simulink model "Modes_Serial"  (R2022b)
settings: Solver=FixedStepAuto  StartTime=0.0  StopTime=10.0  FixedStep=1e-3  RelTol=1e-3  EnableMultiTasking=on
undefined symbols (not defined in the file): A0, A1, D0, D1, D10, D11, D12, D13, D2, D3, D4, D5, D6, D7, D8, D9, PTA0, PTA1, PTA2, PTB2, PTB23, PTB3, PTB9, PTC16, PTC17, PTC2, PTC3, PTC4, PTD0, PTD1, PTD2, PTD3
libraries: etargetslib x22, frdmk64flib x21
settings Model: ExtModeTrigDuration=5  Creator=haotianxue  LastModifiedBy=kavem
settings OptimizationCC: EnhancedBackFolding=on  PassReuseOutputArgsAs=Individual arguments  ZeroExternalMemoryAtStartup=off  ZeroInternalMemoryAtStartup=off  MaxStackSize=64  OptimizeBlockOrder=speed  DifferentSizesBufferReuse=on  OptimizationCustomize=off  EfficientTunableParamExpr=on
settings DebuggingCC: ParameterTunabilityLossMsg=error  UnconnectedInputMsg=warning  UnconnectedOutputMsg=warning  UnconnectedLineMsg=warning
settings HardwareCC: ProdBitPerPointer=32  ProdBitPerSizeT=32  ProdBitPerPtrDiffT=32  ProdLargestAtomicInteger=Long  ProdLargestAtomicFloat=Double  ProdWordSize=32  ProdHWDeviceType=ARM Compatible->ARM Cortex
settings ModelReferenceCC: EnableRefExpFcnMdlSchedulingChecks=on
settings SFSimCC: MATLABDynamicMemAlloc=off
settings RTWCC: Description=Embedded Coder  SystemTargetFile=ert.tlc  HardwareBoard=NXP FRDM-K64F  TLCOptions="-aInlineSetEventsForThisBaseRateFcn=TLC_FALSE -aSuppressMultiTaskScheduler=TLC_FALSE  -aRateBasedStepFcn=0"  TemplateMakefile=ert_default_tmf  Toolchain=GNU Tools for ARM Embedded Processors  DLArmComputeVersion=19.05
settings CodeAppCC: ForceParamTrailComments=on  IgnoreCustomStorageClasses=off  OperatorAnnotations=on  SimulinkDataObjDesc=on  SFDataObjDesc=on  InsertBlockDesc=on
settings ERTTargetCC: ExtModeTransport=4  ExtModeMexFile=sendToCommService

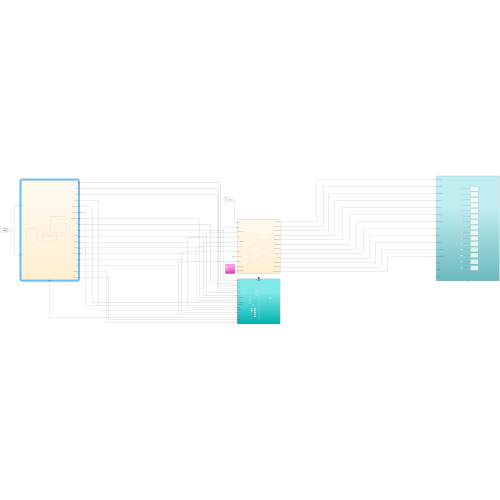
[thumbnail: Simulink's stored preview of the top-level diagram]
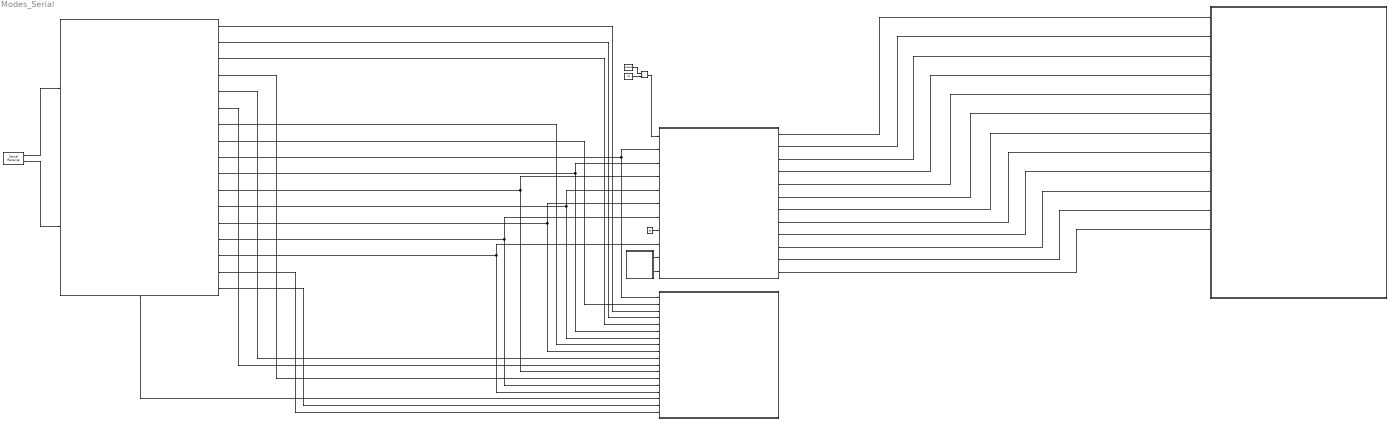
== system Modes_Serial ==
  COM_IN : Stateflow chart  TreatAsAtomicUnit=on
      settings: PortSchema="{\"entries\":[{\"content\":{\"sides\":[{\"content\":{\"connectorIds\":[\"In1\",\"In2\"]},\"type\":\"ConnectorPlacement.EquallySpacedRectSide\",\"uuid\":\"8214c444-1de1-4d31-bdd0-fdf28bd65edf\"},{\"content\":{\"connectorIds\":[\"Out1\",\"Out2\",\"Out3\",\"Out4\",\"Out5\",\"Out6\",\"Out7\",\"Out8\",\"Out9\",\"Out10\",\"Out11\",\"Out12\",\"Out13\",\"Out14\",\"Out15\",\"Out16\",\"Out17\"],\"side\":\"RIGHT\"},\"type\":\"ConnectorPlacement.EquallySpacedRectSide\",\"uuid\":\"fd4b820b-d988-4087-aa44-295b159a4f83\"},{\"content\":{\"connectorIds\":[],\"side\":\"TOP\"},\"type\":\"ConnectorPlacement.EquallySpacedRectSide\",\"uuid\":\"9cb3f67b-9bed-4d96-a295-eb351e913ea4\"},{\"content\":{\"connectorIds\":[\"Out18\"],\"side\":\"BOTTOM\"},\"type\":\"ConnectorPlacement.EquallySpacedRectSide\",\"uuid\":\"87181d9a-e9d0-4f8b-bc10-3b203b2fc102\"}]},\"type\":\"ConnectorPlacement.EquallySpacedConnector\",\"uuid\":\"39350b03-ea46-4b33-9d0b-af5e3b674f3a\"}],\"packageUris\":[\"http://schema.mathworks.com/mf0/Connector/R2020b\"],\"version\":\"1.0\"}"
  Chart : Stateflow chart  TreatAsAtomicUnit=on
  Constant : Constant  Value=60000
  Constant1 : Constant  Value=60
  Constant2 : Constant  Value=80
  Divide : Product  Inputs=*/
  Function-Call Subsystem1 : Subsystem  TreatAsAtomicUnit=on
  Outputs2 : Subsystem
  Serial Receive1 : frdmk64flib/Serial Receive  SCIModule=0  Baudrate=uint32(9600)  Parity=None  StopBits=1  HardwareFlowControl=None  ByteOrder=LittleEndian  DataType=uint8  DataLength=36  BlockingMode=off  OutputStatus=on  SampleTime=-1
  Subsystem : Subsystem
  wires:
  Chart/2(ATR_PACE_CTRL) -> Outputs2/2(ATR_PACE_CTRL)
  Chart/11(ATR_CMP_REF_PWM) -> Outputs2/11(ATR_CMP_REF_PWM)
  Chart/7(VENT_PACE_CTRL) -> Outputs2/7("VENT_PACE_CTRL ")
  Chart/10(FRONTEND_CTRL) -> Outputs2/10(FRONTEND_CTRL)
  Chart/8(Z_ATR_CTRL) -> Outputs2/8("Outputs ")
  Chart/9(Z_VENT_CTRL) -> Outputs2/9(Outputs 1)
  Chart/6(VENT_GND_CTRL) -> Outputs2/6("VENT_GND_CTRL ")
  Chart/5(PACING_REF_PWM) -> Outputs2/5(PACING_REF_PWM)
  Constant/1 -> Divide/1
  Chart/12(VENT_CMP_REF_PWM) -> Outputs2/12(VENT_CMP_REF_PWM)
  Chart/1(ATR_GND_CTRL) -> Outputs2/1(ATR_GND_CTRL)
  Chart/3(PACE_CHARGE_CTRL) -> Outputs2/3(PACE_CHARGE_CTRL)
  Chart/4(PACE_GND_CTRL) -> Outputs2/4("PACE_GND_CTRL ")
  Serial Receive1/1 -> COM_IN/1(rxdata)
  Serial Receive1/2 -> COM_IN/2(status)
  COM_IN/1(LRL_b) -> Function-Call Subsystem1/3(LRL_b)  "LRL"
  COM_IN/2(URL_b) -> Function-Call Subsystem1/4(URL_b)  "URL"
  COM_IN/3(MSR_b) -> Function-Call Subsystem1/5(MSR_b)  "MSR"
  COM_IN/4(ACT_THRES_b) -> Function-Call Subsystem1/13(ACT_THRES)  "THRESHOLD"
  COM_IN/5(REACTION_TIME_b) -> Function-Call Subsystem1/10(REACTION_TIME)  "REACTION"
  COM_IN/6(RECOVERY_TIME_b) -> Function-Call Subsystem1/11(RECOVERY_TIME)  "RECOVERY"
  COM_IN/7(RESPONSE_FACTOR_b) -> Function-Call Subsystem1/8(RESPONSE_FACTOR)  "RESPONSE"
  COM_IN/8(RA_on) -> Function-Call Subsystem1/2(RA_on)  "RA_ON"
  COM_IN/9(mode) -> Chart/2(MODE), Function-Call Subsystem1/1(mode)  "MODE"
  COM_IN/10(ATR_PW_b) -> Chart/3(ATR_PULSE_WIDTH), Function-Call Subsystem1/6(ATR_PW)  "ATR_PW"
  COM_IN/11(ATR_AMP_b) -> Chart/4(ATR_Amp), Function-Call Subsystem1/12(ATR_AMP)  "ATR_AMP"
  COM_IN/12(VENT_PW_b) -> Chart/5(VENT_PULSE_WIDTH), Function-Call Subsystem1/7(VENT_PW)  "VENT_PW"
  COM_IN/13(VENT_AMP_b) -> Chart/6(VENT_Amp), Function-Call Subsystem1/9(VENT_AMP)  "VENT_AMP"
  COM_IN/14(ARP_b) -> Chart/7(ATR_RP), Function-Call Subsystem1/14(ARP)  "ATR_RP"
  COM_IN/15(VRP_b) -> Chart/9(VENT_RP), Function-Call Subsystem1/15(VRP)  "VENT_RP"
  Constant2/1 -> Chart/8(Sample_Amp)
  Subsystem/1(ATR) -> Chart/10(ATR_CMP_DETECT)
  Subsystem/2(VENT) -> Chart/11(VENT_CMP_DETECT)
  COM_IN/18(egram) -> Function-Call Subsystem1/16(egram)
  Divide/1 -> Chart/1(PERIOD)
  COM_IN/16(ATR_SENS_b) -> Function-Call Subsystem1/18(ATR_sens)
  COM_IN/17(VENT_SENS_b) -> Function-Call Subsystem1/17(VENT_sens)
  Constant1/1 -> Divide/2

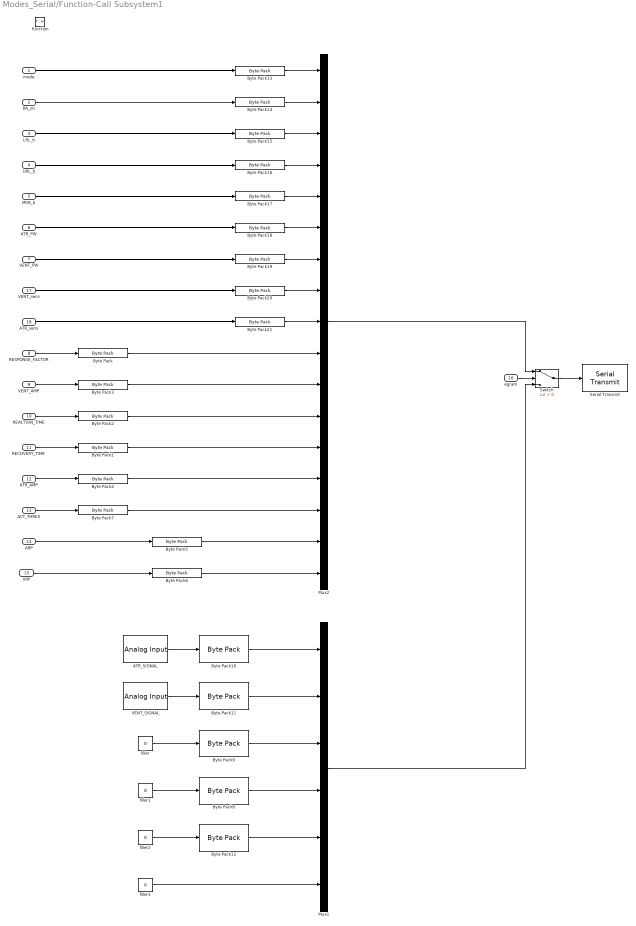
== system Modes_Serial/Function-Call Subsystem1 ==
  mode : Inport
  RA_on : Inport  Port=2
  LRL_b : Inport  Port=3
  URL_b : Inport  Port=4
  MSR_b : Inport  Port=5
  ATR_PW : Inport  Port=6
  VENT_PW : Inport  Port=7
  RESPONSE_FACTOR : Inport  Port=8
  VENT_AMP : Inport  Port=9
  REACTION_TIME : Inport  Port=10
  RECOVERY_TIME : Inport  Port=11
  ATR_AMP : Inport  Port=12
  ACT_THRES : Inport  Port=13
  ARP : Inport  Port=14
  VRP : Inport  Port=15
  egram : Inport  Port=16
  VENT_sens : Inport  Port=17
  ATR_sens : Inport  Port=18
  function : TriggerPort  TriggerType=function-call  IsSimulinkFunction=on  FunctionName=send_paramsss  VariantControl=(inherit)
  ATR_SIGNAL : frdmk64flib/Analog Input  Whichpin=PTB2 (A0)  SampleTime=-1
  Byte Pack{,1..4,7,12} (7 alike) : etargetslib/Byte Pack  datatypes={'single'}  byteAlign=1
  Byte Pack{8..11} (4 alike) : etargetslib/Byte Pack  datatypes={'double'}  byteAlign=1
  Byte Pack{13..21} (9 alike) : etargetslib/Byte Pack  datatypes={'uint8'}  byteAlign=1
  Byte Pack5 : etargetslib/Byte Pack  datatypes={'uint16'}  byteAlign=1
  Byte Pack6 : etargetslib/Byte Pack  datatypes={'uint16'}  byteAlign=1
  Mux1 : Mux  Inputs=6
  Mux2 : Mux  Inputs=17
  Serial Transmit : frdmk64flib/Serial Transmit  SCIModule=0  Baudrate=uint32(9600)  Parity=None  StopBits=1  HardwareFlowControl=None  ByteOrder=LittleEndian  BlockingMode=on  OutputStatus=off
  Switch : Switch  Criteria=u2 > Threshold  SaturateOnIntegerOverflow=off  InputSameDT=off
  VENT_SIGNAL : frdmk64flib/Analog Input  Whichpin=PTB3 (A1)  SampleTime=-1
  filler : Constant  Value=0  OutDataTypeStr=double
  filler1 : Constant  Value=0  OutDataTypeStr=double
  filler2 : Constant  Value=0  OutDataTypeStr=single
  filler3 : Constant  Value=0  OutDataTypeStr=uint8
  wires:
  VENT_sens/1 -> Byte Pack20/1
  Byte Pack/1 -> Mux2/10
  Byte Pack1/1 -> Mux2/13
  Byte Pack2/1 -> Mux2/12
  Byte Pack3/1 -> Mux2/11
  Byte Pack4/1 -> Mux2/14
  Byte Pack5/1 -> Mux2/16
  Byte Pack6/1 -> Mux2/17
  mode/1 -> Byte Pack13/1
  RA_on/1 -> Byte Pack14/1
  LRL_b/1 -> Byte Pack15/1
  URL_b/1 -> Byte Pack16/1
  MSR_b/1 -> Byte Pack17/1
  ATR_PW/1 -> Byte Pack18/1
  VENT_PW/1 -> Byte Pack19/1
  RESPONSE_FACTOR/1 -> Byte Pack/1
  VENT_AMP/1 -> Byte Pack3/1
  REACTION_TIME/1 -> Byte Pack2/1
  RECOVERY_TIME/1 -> Byte Pack1/1
  ATR_AMP/1 -> Byte Pack4/1
  Byte Pack7/1 -> Mux2/15
  ACT_THRES/1 -> Byte Pack7/1
  ARP/1 -> Byte Pack5/1
  Switch/1 -> Serial Transmit/1
  egram/1 -> Switch/2
  Mux2/1 -> Switch/1
  ATR_SIGNAL/1 -> Byte Pack10/1
  VENT_SIGNAL/1 -> Byte Pack11/1
  Mux1/1 -> Switch/3
  Byte Pack10/1 -> Mux1/1
  Byte Pack11/1 -> Mux1/2
  Byte Pack8/1 -> Mux1/4
  Byte Pack9/1 -> Mux1/3
  filler/1 -> Byte Pack9/1
  filler1/1 -> Byte Pack8/1
  Byte Pack12/1 -> Mux1/5
  filler2/1 -> Byte Pack12/1
  filler3/1 -> Mux1/6
  Byte Pack13/1 -> Mux2/1
  Byte Pack14/1 -> Mux2/2
  Byte Pack15/1 -> Mux2/3
  Byte Pack16/1 -> Mux2/4
  Byte Pack17/1 -> Mux2/5
  Byte Pack18/1 -> Mux2/6
  Byte Pack19/1 -> Mux2/7
  Byte Pack20/1 -> Mux2/8
  Byte Pack21/1 -> Mux2/9
  VRP/1 -> Byte Pack6/1
  ATR_sens/1 -> Byte Pack21/1

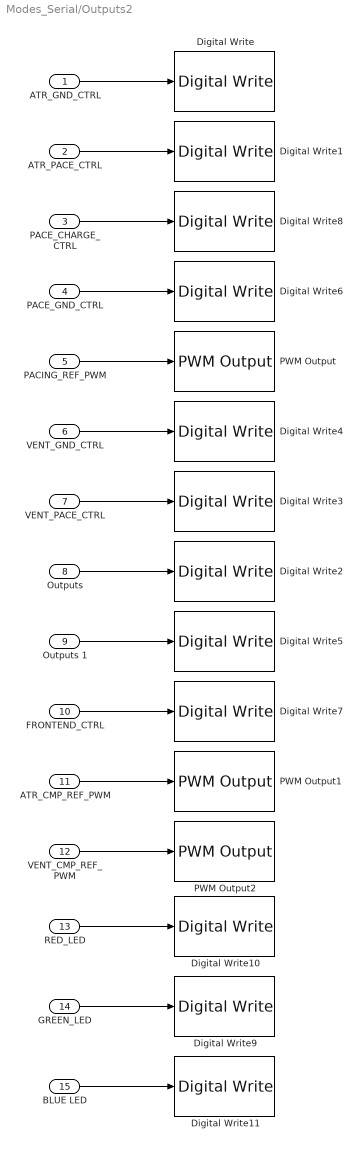
== system Modes_Serial/Outputs2 ==
  ATR_GND_CTRL : Inport
  ATR_PACE_CTRL : Inport  Port=2
  PACE_CHARGE_CTRL : Inport  Port=3
  "PACE_GND_CTRL " : Inport  Port=4
  PACING_REF_PWM : Inport  Port=5
  "VENT_GND_CTRL " : Inport  Port=6
  "VENT_PACE_CTRL " : Inport  Port=7
  "Outputs " : Inport  Port=8
  Outputs 1 : Inport  Port=9
  FRONTEND_CTRL : Inport  Port=10
  ATR_CMP_REF_PWM : Inport  Port=11
  VENT_CMP_REF_PWM : Inport  Port=12
  RED_LED : Inport  Port=13
  GREEN_LED : Inport  Port=14
  BLUE LED : Inport  Port=15
  Digital Write : frdmk64flib/Digital Write  Whichpin=PTD2 (D11)
  Digital Write1 : frdmk64flib/Digital Write  Whichpin=PTA0 (D8)
  Digital Write10 : frdmk64flib/Digital Write  Whichpin=RED_LED
  Digital Write11 : frdmk64flib/Digital Write  Whichpin=BLUE_LED
  Digital Write2 : frdmk64flib/Digital Write  Whichpin=PTB23 (D4)
  Digital Write3 : frdmk64flib/Digital Write  Whichpin=PTC4 (D9)
  Digital Write4 : frdmk64flib/Digital Write  Whichpin=PTD3 (D12)
  Digital Write5 : frdmk64flib/Digital Write  Whichpin=PTC3 (D7)
  Digital Write6 : frdmk64flib/Digital Write  Whichpin=PTD0 (D10)
  Digital Write7 : frdmk64flib/Digital Write  Whichpin=PTD1 (D13)
  Digital Write8 : frdmk64flib/Digital Write  Whichpin=PTB9 (D2)
  Digital Write9 : frdmk64flib/Digital Write  Whichpin=GREEN_LED
  PWM Output : frdmk64flib/PWM Output  Whichpin=PTA2 (D5)  InitialFrequency=2000  InitialDutyCycle=0
  PWM Output1 : frdmk64flib/PWM Output  Whichpin=PTC2 (D6)  InitialFrequency=2000  InitialDutyCycle=0
  PWM Output2 : frdmk64flib/PWM Output  Whichpin=PTA1 (D3)  InitialFrequency=2000  InitialDutyCycle=0
  wires:
  ATR_GND_CTRL/1 -> Digital Write/1
  ATR_PACE_CTRL/1 -> Digital Write1/1
  PACE_CHARGE_CTRL/1 -> Digital Write8/1
  RED_LED/1 -> Digital Write10/1
  GREEN_LED/1 -> Digital Write9/1
  BLUE LED/1 -> Digital Write11/1
  "PACE_GND_CTRL "/1 -> Digital Write6/1
  PACING_REF_PWM/1 -> PWM Output/1
  "VENT_GND_CTRL "/1 -> Digital Write4/1
  "VENT_PACE_CTRL "/1 -> Digital Write3/1
  "Outputs "/1 -> Digital Write2/1
  Outputs 1/1 -> Digital Write5/1
  FRONTEND_CTRL/1 -> Digital Write7/1
  ATR_CMP_REF_PWM/1 -> PWM Output1/1
  VENT_CMP_REF_PWM/1 -> PWM Output2/1

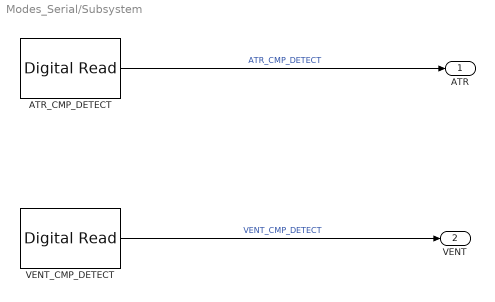
== system Modes_Serial/Subsystem ==
  ATR_CMP_DETECT : frdmk64flib/Digital Read  Whichpin=PTC16 (D0)  SampleTime=-1
  VENT_CMP_DETECT : frdmk64flib/Digital Read  Whichpin=PTC17 (D1)  SampleTime=-1
  ATR : Outport
  VENT : Outport  Port=2
  wires:
  VENT_CMP_DETECT/1 -> VENT/1  "VENT_CMP_DETECT"
  ATR_CMP_DETECT/1 -> ATR/1  "ATR_CMP_DETECT"

== stateflow chart Modes_Serial/Chart ==
  state Identify_Mode_Path1
    entry:
    % MODE = 1 (AOO)
    % MODE = 2 (AAI)
    % MODE = 3 (VOO)
    % MODE = 4 (VVI)
    %
    %pacemaker disconnected
    %stop sensing
    PACE_CHARGE_CTRL = LOW
    VENT_PACE_CTRL = LOW
    ATR_PACE_CTRL = LOW
    PACE_GND_CTRL = LOW
    ATR_GND_CTRL = LOW
    VENT_GND_CTRL = LOW
    Z_ATR_CTRL = LOW
    Z_VENT_CTRL = LOW
    FRONTEND_CTRL = LOW
  state AOO1
    entry:
    %Charge primary capcitor C22
    ATR_PACE_CTRL=LOW
    PACING_REF_PWM = 20*ATR_Amp
    PACE_CHARGE_CTRL = HIGH
    %Discharge block capacitor C21
    PACE_GND_CTRL = HIGH
    ATR_GND_CTRL = HIGH
    %use LED  to verify state
  state AOO_ATR_PULSE1
    entry:
    %Discharge C22 primary capacitor
    %Charge C21 block capacitor
    PACE_CHARGE_CTRL = LOW
    PACE_GND_CTRL = HIGH
    ATR_PACE_CTRL = HIGH
    ATR_GND_CTRL = LOW
    PACING_REF_PWM = 20*ATR_Amp
    %use LED  to verify state
  state AAI_ATR_PULSE1
    entry:
    %sensing OFF
    FRONTEND_CTRL = LOW
    %Discharge C22 primary capacitor
    %Charge C21 block capacitor
    PACE_CHARGE_CTRL = LOW
    PACE_GND_CTRL = HIGH
    ATR_PACE_CTRL = HIGH
    ATR_GND_CTRL = LOW
    PACING_REF_PWM = 20*ATR_Amp
    %use LED  to verify state
  state AAI1
    entry:
    %sensing ON
    FRONTEND_CTRL = HIGH
    %Charge primary capcitor C22
    ATR_PACE_CTRL=LOW
    PACING_REF_PWM = 20*ATR_Amp
    PACE_CHARGE_CTRL = HIGH
    %Discharge block capacitor C21
    PACE_GND_CTRL = HIGH
    ATR_GND_CTRL = HIGH
    ATR_CMP_REF_PWM = Sample_Amp
    %use LED  to verify state
  state VOO1
    entry:
    %Charge primary capcitor C22
    VENT_PACE_CTRL=LOW
    PACING_REF_PWM = 20*VENT_Amp
    PACE_CHARGE_CTRL = HIGH
    %Discharge block capacitor C21
    PACE_GND_CTRL = HIGH
    VENT_GND_CTRL = HIGH
    %use LED  to verify state
  state VOO_VENT_PULSE1
    entry:
    %Discharge C22 primary capacitor
    %Charge C21 block capacitor
    PACE_CHARGE_CTRL = LOW
    PACE_GND_CTRL = HIGH
    VENT_GND_CTRL = LOW
    VENT_PACE_CTRL  = HIGH
    PACING_REF_PWM = 20*VENT_Amp
    %use LED  to verify state
  state VVI1
    entry:
    %sensing ON
    FRONTEND_CTRL = HIGH
    %Charge primary capcitor C22
    VENT_PACE_CTRL= LOW
    PACING_REF_PWM = 20*VENT_Amp
    PACE_CHARGE_CTRL = HIGH
    %Discharge block capacitor C21
    PACE_GND_CTRL = HIGH
    VENT_PACE_CTRL = LOW
    VENT_GND_CTRL = HIGH
    VENT_CMP_REF_PWM = Sample_Amp
    %use LED  to verify state
  state VVI_VENT_PULSE1
    %sensing OFF
    FRONTEND_CTRL = LOW
    %Discharge C22 primary capacitor
    %Charge C21 block capacitor
    PACE_CHARGE_CTRL = LOW
    PACE_GND_CTRL = HIGH
    VENT_GND_CTRL = LOW
    VENT_PACE_CTRL  = HIGH
    PACING_REF_PWM = 20*VENT_Amp
    %use LED  to verify state
  (default) -> Identify_Mode_Path1
  AOO1 -> AOO_ATR_PULSE1 : after(PERIOD - ATR_PULSE_WIDTH,msec)
  Identify_Mode_Path1 -> AOO1 [order 1] : [MODE == 1]
  AOO_ATR_PULSE1 -> AOO1 : after(ATR_PULSE_WIDTH,msec)
  AAI_ATR_PULSE1 -> AAI1 : after(ATR_PULSE_WIDTH,msec)
  Identify_Mode_Path1 -> AAI1 [order 2] : [MODE == 2]
  AAI1 -> (junction 113)
  (junction 113) -> AAI_ATR_PULSE1 [order 1] : after(PERIOD - ATR_PULSE_WIDTH,msec)[ATR_CMP_DETECT == LOW]
  (junction 113) -> AAI1 [order 2] : after(ATR_RP, msec)[ATR_CMP_DETECT == HIGH]
  VOO1 -> VOO_VENT_PULSE1 : after(PERIOD - VENT_PULSE_WIDTH,msec)
  Identify_Mode_Path1 -> VOO1 [order 3] : [MODE == 3]
  VOO_VENT_PULSE1 -> VOO1 : after(VENT_PULSE_WIDTH,msec)
  VVI_VENT_PULSE1 -> VVI1 : after(VENT_PULSE_WIDTH,msec)
  Identify_Mode_Path1 -> VVI1 [order 4] : [MODE == 4]
  VVI1 -> (junction 119)
  (junction 119) -> VVI_VENT_PULSE1 [order 1] : after(PERIOD - VENT_PULSE_WIDTH,msec)[VENT_CMP_DETECT == LOW]
  (junction 119) -> VVI1 [order 2] : after(VENT_RP, msec)[VENT_CMP_DETECT == HIGH]
  data: PERIOD input; MODE input; ATR_PULSE_WIDTH input; ATR_Amp input; VENT_PULSE_WIDTH input; VENT_Amp input; ATR_RP input; Sample_Amp input; VENT_RP input; ATR_CMP_DETECT input; VENT_CMP_DETECT input; HIGH local =1; LOW local =0; ATR_GND_CTRL output; ATR_PACE_CTRL output; PACE_CHARGE_CTRL output; PACE_GND_CTRL output; PACING_REF_PWM output; VENT_GND_CTRL output; VENT_PACE_CTRL output; Z_ATR_CTRL output; Z_VENT_CTRL output; FRONTEND_CTRL output; ATR_CMP_REF_PWM output; VENT_CMP_REF_PWM output

== stateflow chart Modes_Serial/COM_IN ==
  state SET_PARAM
    entry:
    %red_en = rxdata(3);
    %green_en =  rxdata(4);
    %blue_en = rxdata(5);
    %off_time = typecast(rxdata(6:9), 'single');
    %switch_time = typecast(rxdata(10:11), 'uint16');
    egram = 1;
    mode = rxdata(3)
    RA_on = rxdata(4);
    LRL_b = rxdata(5)
    URL_b = rxdata(6)
    MSR_b = rxdata(7)
    ATR_PW_b = rxdata(8);
    VENT_PW_b = rxdata(9);
    VENT_SENS_b = rxdata(10);
    ATR_SENS_b = rxdata(11);
    RESPONSE_FACTOR_b = typecast(rxdata(12:15), 'single');
    VENT_AMP_b = typecast(rxdata(16:19), 'single');
    REACTION_TIME_b = typecast(rxdata(20:23), 'single');
    RECOVERY_TIME_b = typecast(rxdata(24:27), 'single');
    ATR_AMP_b = typecast(rxdata(28:31), 'single');
    ACT_THRES_b = typecast(rxdata(32:35), 'single');
    ARP_b = typecast(rxdata(36:37), 'uint16');
    VRP_b = typecast(rxdata(38:39), 'uint16');
  state INITIAL
    entry:
    %red_en = 1;
    %green_en = 1;
    %blue_en = 1;
    %off_time = 0.5;
    %switch_time = 200;
    URL_b = uint8(120);
    LRL_b = uint8(60);
    MSR_b = uint8(120);
    mode = uint8(1);
    RA_on = uint8(0);
    ATR_PW_b = uint8(5);
    ATR_AMP_b = single(1);
    VENT_PW_b = uint8(5);
    VENT_AMP_b = single(3.75);
    ARP_b = uint16(250);
    VRP_b = uint16(350);
    VENT_SENS_b = uint8(2);
    ATR_SENS_b = uint8(1);
    REACTION_TIME_b = single(30.0);
    RECOVERY_TIME_b = single(5.0);
    RESPONSE_FACTOR_b = single(8.0);
    ACT_THRES_b = single(1.2);
  state SEND_EGRAM
    entry:
    egram = 0
    send_paramsss()
  state STANDBY
    entry:
    egram = 1
  state ECHO_PARAM
    entry:
    send_paramsss();
  (default) -> INITIAL
  SET_PARAM -> STANDBY
  (junction 15) -> SET_PARAM [order 2] : [rxdata(2)==hex2dec('55')]
  (junction 14) -> STANDBY [order 2]
  INITIAL -> STANDBY
  STANDBY -> (junction 14) : [status==0]
  (junction 14) -> (junction 15) [order 1] : [rxdata(1)==hex2dec('16')]
  (junction 15) -> SEND_EGRAM [order 1] : [rxdata(2)==hex2dec('47')]
  SEND_EGRAM -> STANDBY
  (junction 15) -> ECHO_PARAM [order 3] : [rxdata(2)==hex2dec('22')]
  ECHO_PARAM -> STANDBY
  data: LRL_b output uint8; URL_b output uint8; MSR_b output uint8; rxdata input uint8; status input uint8; ACT_THRES_b output single; REACTION_TIME_b output single; RECOVERY_TIME_b output single; RESPONSE_FACTOR_b output single; RA_on output uint8; mode output uint8; ATR_PW_b output uint8; ATR_AMP_b output single; VENT_PW_b output uint8; VENT_AMP_b output single; ARP_b output uint16; VRP_b output uint16; ATR_SENS_b output uint8; VENT_SENS_b output uint8; egram output
